simulink model "Frontier40GAPOUT"  (R2015b)
settings: Solver=FixedStepAuto  StartTime=0.0  StopTime=inf  FixedStep=0.1  RelTol=1e-3
values from neighbouring files (symbols this model uses):
  GAPS = []    [ASS.mat]    (also in ENDOFFNC.mat = [26 13 7.5 29.5 29 8.5 29.5 26 30 5.5 34 5 ... (988 elements; FrontierA50GAPSPLOT.m = GAPS_found(i,:); GAPPIE.mat = [26 13 7.5 29.5 29 8.5 29.5 26 30 5.5 34 5 ... (988 elements; HERE.mat = [26 13 7.5 29.5 29 8.5 29.5 26 30 5.5 34 5 ... (988 elements)
  map = [2 0 0 0 0 0 0 0 0 0 0 0 ... (1600 elements, 40x40)]    [INfShitt.mat]
  Method = 1    [ASS.mat]    (also in ENDOFFNC.mat = 0; FrontierA50GAPSPLOT.m = u(end,7); GAPPIE.mat = 0; HERE.mat = 0)
undefined symbols (not defined in the file or in its folder): Data, Data_SL_Info, X, Y, Z
libraries: robotlib x17
settings Model: Creator=einar  LastModifiedBy=einar

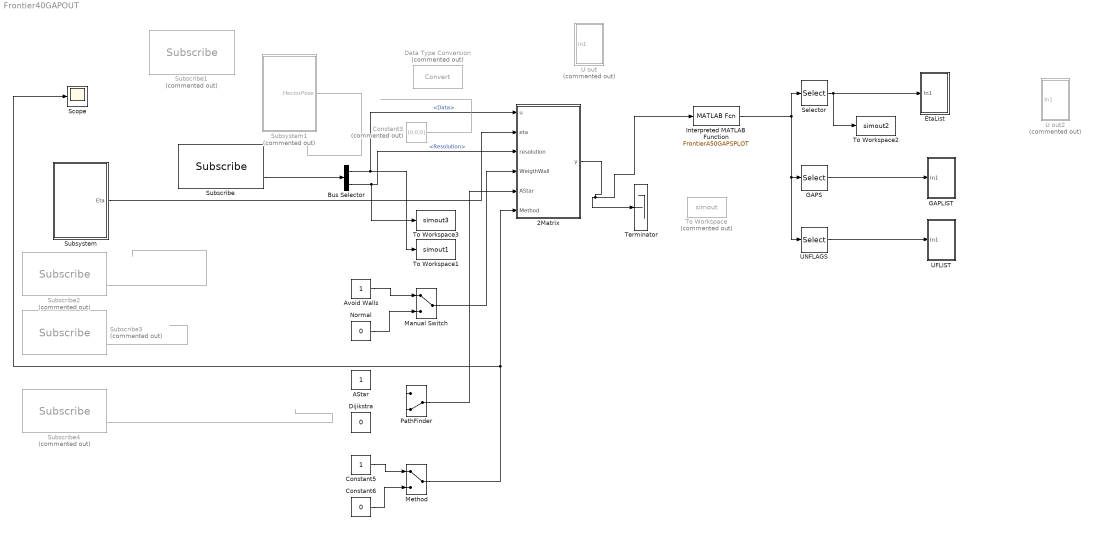
== system Frontier40GAPOUT ==
  2Matrix : MATLAB Function  TreatAsAtomicUnit=on
  AStar : Constant
  Avoid Walls : Constant
  Bus Selector : BusSelector  OutputSignals=Data,Info.Resolution
  Constant3 : Constant  Commented=on  Value=[0;0;0]
  Constant5 : Constant
  Constant6 : Constant  Value=0
  Data Type Conversion : DataTypeConversion  Commented=on
  Dijikstra : Constant  Value=0
  EtaList : Subsystem
  GAPLIST : Subsystem
  GAPS : Selector  InputPortWidth=768  IndexOptions=Index vector (dialog)  Indices=[257:512]  OutputSizes=1
  Interpreted MATLAB Function : MATLABFcn  MATLABFcn=FrontierA50GAPSPLOT  OutputDimensions=768
  Manual Switch : ManualSwitch
  Method : ManualSwitch
  Normal : Constant  Value=0
  PathFinder : ManualSwitch  CurrentSetting=0
  Scope : Scope
  Selector : Selector  InputPortWidth=768  IndexOptions=Index vector (dialog)  Indices=[1:256]  OutputSizes=1
  Subscribe : robotlib/Subscribe  SourceLibraryInfo=This block requires Robotics System Toolbox  topicSource=Select from ROS network  topic=/map  messageType=nav_msgs/OccupancyGrid  sampleTime=0.5  messageQueueLength=1
  Subscribe1 : robotlib/Subscribe  Commented=on  SourceLibraryInfo=This block requires Robotics System Toolbox  topicSource=Select from ROS network  topic=/ExploredOccupancyGrid  messageType=nav_msgs/OccupancyGrid  sampleTime=0.5  messageQueueLength=1
  Subscribe2 : robotlib/Subscribe  Commented=on  SourceLibraryInfo=This block requires Robotics System Toolbox  topicSource=Specify your own  topic=/AStar  messageType=std_msgs/Bool  sampleTime=-1  messageQueueLength=1
  Subscribe3 : robotlib/Subscribe  Commented=on  SourceLibraryInfo=This block requires Robotics System Toolbox  topicSource=Specify your own  topic=/WeighWall  messageType=std_msgs/Bool  sampleTime=-1  messageQueueLength=1
  Subscribe4 : robotlib/Subscribe  Commented=on  SourceLibraryInfo=This block requires Robotics System Toolbox  topicSource=Specify your own  topic=/Method  messageType=std_msgs/Bool  sampleTime=-1  messageQueueLength=1
  Subsystem : Subsystem
  Subsystem1 : Subsystem  Commented=on
  Terminator : Terminator
  To Workspace : ToWorkspace  Commented=on  VariableName=simout  SaveFormat=Timeseries  SampleTime=-1
  To Workspace1 : ToWorkspace  VariableName=simout1  SaveFormat=Timeseries  SampleTime=-1
  To Workspace2 : ToWorkspace  VariableName=simout2  SaveFormat=Timeseries  SampleTime=-1
  To Workspace3 : ToWorkspace  VariableName=simout3  SaveFormat=Timeseries  SampleTime=-1
  U out : Subsystem  Commented=on
  U out2 : Subsystem  Commented=on
  "UFLIST " : Subsystem
  UNFLAGS : Selector  InputPortWidth=768  IndexOptions=Index vector (dialog)  Indices=[513:768]  OutputSizes=1
  wires:
  Subscribe/2 -> Bus Selector/1
  Bus Selector/1 -> To Workspace1/1, 2Matrix/1(u)  "<Data>"
  2Matrix/1(y) -> Interpreted MATLAB Function/1, Terminator/1
  Subsystem/1(Eta) -> 2Matrix/2(eta)
  Subsystem1/1("HectorPose ") -> ?
  Bus Selector/2 -> To Workspace3/1, 2Matrix/3(resolution)  "<Resolution>"
  Interpreted MATLAB Function/1 -> UNFLAGS/1, GAPS/1, Selector/1
  ? -> U out/1(In1)
  Subscribe2/2 -> ?
  Subscribe3/2 -> ?
  Subscribe4/2 -> ?
  Manual Switch/1 -> 2Matrix/4(WeigthWall)
  Constant3/1 -> ?
  Avoid Walls/1 -> Manual Switch/1
  Normal/1 -> Manual Switch/2
  Constant5/1 -> Method/1
  Constant6/1 -> Method/2
  PathFinder/1 -> 2Matrix/5(AStar)
  Method/1 -> 2Matrix/6(Method), Scope/1
  Selector/1 -> EtaList/1(In1), To Workspace2/1
  GAPS/1 -> GAPLIST/1(In1)
  UNFLAGS/1 -> "UFLIST "/1(In1)

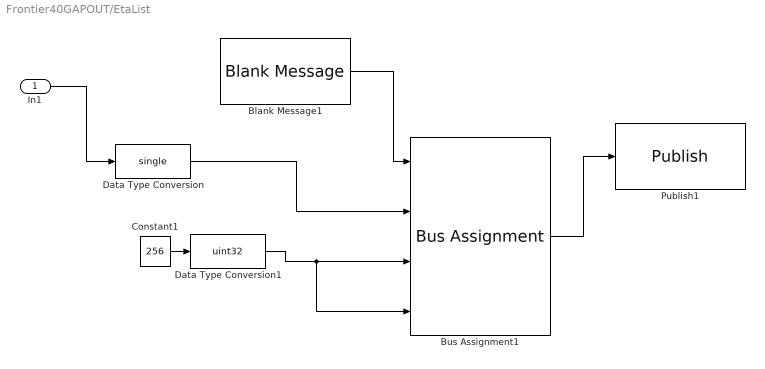
== system Frontier40GAPOUT/EtaList ==
  In1 : Inport
  Blank Message1 : robotlib/Blank Message  SourceLibraryInfo=This block requires Robotics System Toolbox  messageType=std_msgs/Float32MultiArray  SampleTime=inf
  Bus Assignment1 : BusAssignment  AssignedSignals=Data,Data_SL_Info.CurrentLength,Data_SL_Info.ReceivedLength
  Constant1 : Constant  Value=256
  Data Type Conversion : DataTypeConversion  OutDataTypeStr=single
  Data Type Conversion1 : DataTypeConversion  OutDataTypeStr=uint32
  Publish1 : robotlib/Publish  SourceLibraryInfo=This block requires Robotics System Toolbox  topicSource=Specify your own  topic=/EtaSetList  messageType=std_msgs/Float32MultiArray  messageQueueLength=1
  wires:
  Constant1/1 -> Data Type Conversion1/1
  Data Type Conversion/1 -> Bus Assignment1/2
  Bus Assignment1/1 -> Publish1/1
  Blank Message1/1 -> Bus Assignment1/1
  Data Type Conversion1/1 -> Bus Assignment1/4, Bus Assignment1/3
  In1/1 -> Data Type Conversion/1

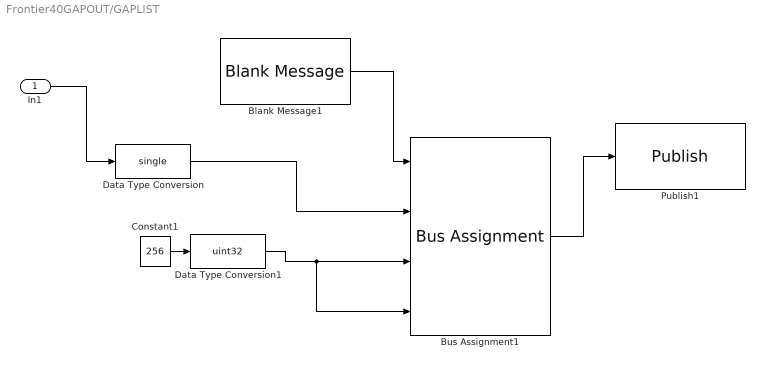
== system Frontier40GAPOUT/GAPLIST ==
  In1 : Inport
  Blank Message1 : robotlib/Blank Message  SourceLibraryInfo=This block requires Robotics System Toolbox  messageType=std_msgs/Float32MultiArray  SampleTime=inf
  Bus Assignment1 : BusAssignment  AssignedSignals=Data,Data_SL_Info.CurrentLength,Data_SL_Info.ReceivedLength
  Constant1 : Constant  Value=256
  Data Type Conversion : DataTypeConversion  OutDataTypeStr=single
  Data Type Conversion1 : DataTypeConversion  OutDataTypeStr=uint32
  Publish1 : robotlib/Publish  SourceLibraryInfo=This block requires Robotics System Toolbox  topicSource=Specify your own  topic=/GAPS  messageType=std_msgs/Float32MultiArray  messageQueueLength=1
  wires:
  In1/1 -> Data Type Conversion/1
  Data Type Conversion1/1 -> Bus Assignment1/3, Bus Assignment1/4
  Blank Message1/1 -> Bus Assignment1/1
  Bus Assignment1/1 -> Publish1/1
  Data Type Conversion/1 -> Bus Assignment1/2
  Constant1/1 -> Data Type Conversion1/1

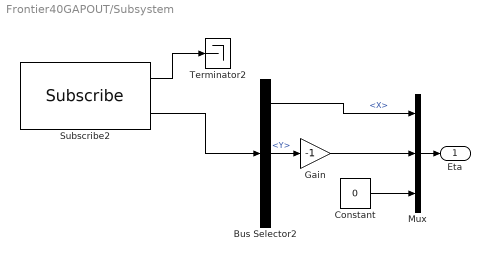
== system Frontier40GAPOUT/Subsystem ==
  Bus Selector2 : BusSelector  OutputSignals=X,Y,Z
  Constant : Constant  Value=0
  Gain : Gain  Gain=-1
  Mux : Mux  Inputs=3
  Subscribe2 : robotlib/Subscribe  SourceLibraryInfo=This block requires Robotics System Toolbox  topicSource=Specify your own  topic=/Eta  messageType=geometry_msgs/Vector3  sampleTime=-1  messageQueueLength=1
  Terminator2 : Terminator
  Eta : Outport
  wires:
  Bus Selector2/1 -> Mux/1  "<X>"
  Subscribe2/2 -> Bus Selector2/1
  Mux/1 -> Eta/1
  Subscribe2/1 -> Terminator2/1
  Bus Selector2/2 -> Gain/1  "<Y>"
  Constant/1 -> Mux/3
  Gain/1 -> Mux/2

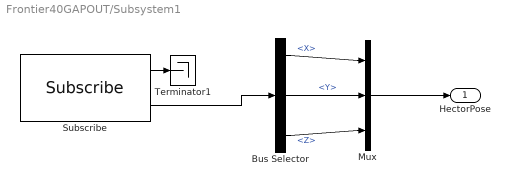
== system Frontier40GAPOUT/Subsystem1 ==
  Bus Selector : BusSelector  OutputSignals=Pose.Pose.Position.X,Pose.Pose.Position.Y,Pose.Pose.Orientation.Z
  Mux : Mux  Inputs=3
  Subscribe : robotlib/Subscribe  SourceLibraryInfo=This block requires Robotics System Toolbox  topicSource=Select from ROS network  topic=/poseupdate  messageType=geometry_msgs/PoseWithCovarianceStamped  sampleTime=-1  messageQueueLength=1
  Terminator1 : Terminator
  "HectorPose " : Outport
  wires:
  Subscribe/2 -> Bus Selector/1
  Subscribe/1 -> Terminator1/1
  Bus Selector/3 -> Mux/3  "<Z>"
  Bus Selector/2 -> Mux/2  "<Y>"
  Bus Selector/1 -> Mux/1  "<X>"
  Mux/1 -> "HectorPose "/1

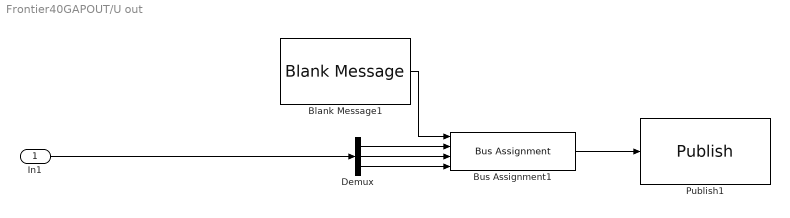
== system Frontier40GAPOUT/U out ==
  In1 : Inport
  Blank Message1 : robotlib/Blank Message  SourceLibraryInfo=This block requires Robotics System Toolbox  messageType=geometry_msgs/Vector3  SampleTime=inf
  Bus Assignment1 : BusAssignment  AssignedSignals=X,Y,Z
  Demux : Demux  Outputs=3
  Publish1 : robotlib/Publish  SourceLibraryInfo=This block requires Robotics System Toolbox  topicSource=Specify your own  topic=/U  messageType=geometry_msgs/Vector3  messageQueueLength=1
  wires:
  Bus Assignment1/1 -> Publish1/1
  Blank Message1/1 -> Bus Assignment1/1
  In1/1 -> Demux/1
  Demux/1 -> Bus Assignment1/2
  Demux/2 -> Bus Assignment1/3
  Demux/3 -> Bus Assignment1/4

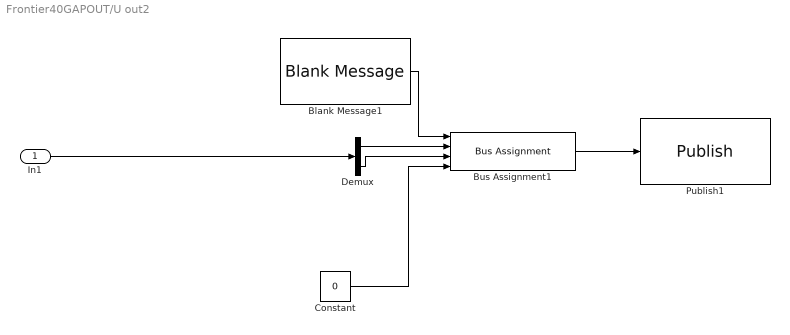
== system Frontier40GAPOUT/U out2 ==
  In1 : Inport
  Blank Message1 : robotlib/Blank Message  SourceLibraryInfo=This block requires Robotics System Toolbox  messageType=geometry_msgs/Vector3  SampleTime=inf
  Bus Assignment1 : BusAssignment  AssignedSignals=X,Y,Z
  Constant : Constant  Value=0
  Demux : Demux  Outputs=2
  Publish1 : robotlib/Publish  SourceLibraryInfo=This block requires Robotics System Toolbox  topicSource=Select from ROS network  topic=/EtaSet  messageType=geometry_msgs/Vector3  messageQueueLength=1
  wires:
  Bus Assignment1/1 -> Publish1/1
  Blank Message1/1 -> Bus Assignment1/1
  In1/1 -> Demux/1
  Demux/1 -> Bus Assignment1/2
  Demux/2 -> Bus Assignment1/3
  Constant/1 -> Bus Assignment1/4

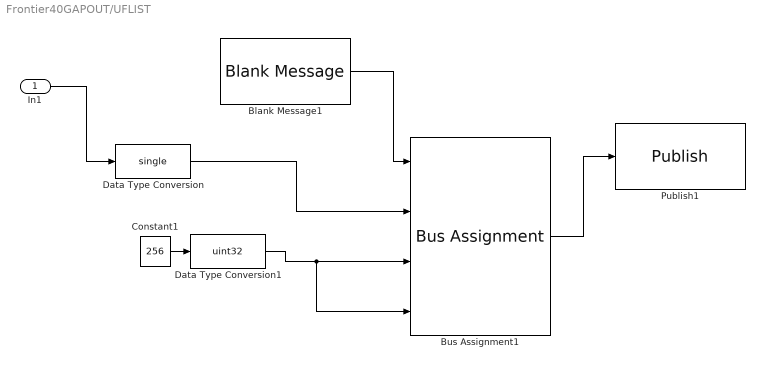
== system Frontier40GAPOUT/UFLIST  ==
  In1 : Inport
  Blank Message1 : robotlib/Blank Message  SourceLibraryInfo=This block requires Robotics System Toolbox  messageType=std_msgs/Float32MultiArray  SampleTime=inf
  Bus Assignment1 : BusAssignment  AssignedSignals=Data,Data_SL_Info.CurrentLength,Data_SL_Info.ReceivedLength
  Constant1 : Constant  Value=256
  Data Type Conversion : DataTypeConversion  OutDataTypeStr=single
  Data Type Conversion1 : DataTypeConversion  OutDataTypeStr=uint32
  Publish1 : robotlib/Publish  SourceLibraryInfo=This block requires Robotics System Toolbox  topicSource=Specify your own  topic=/UNFGAPS  messageType=std_msgs/Float32MultiArray  messageQueueLength=1
  wires:
  Constant1/1 -> Data Type Conversion1/1
  Data Type Conversion/1 -> Bus Assignment1/2
  Bus Assignment1/1 -> Publish1/1
  Blank Message1/1 -> Bus Assignment1/1
  Data Type Conversion1/1 -> Bus Assignment1/4, Bus Assignment1/3
  In1/1 -> Data Type Conversion/1

== matlab function Frontier40GAPOUT/2Matrix ==
  data: u input; y output; eta input; resolution input; WeigthWall input; AStar input; Method input
function y  = fcn(u,eta,resolution,WeigthWall,AStar,Method)
K=length(u)^0.5;
y=zeros(K+1,K);
MAP=zeros(K+1,K)
for i=1:K;
    MAP(i,1:K)=u((i-1)*K+1:i*K);
end
MAP(K+1,1:3)=eta;
MAP(K+1,4)=resolution;
MAP(K+1,5)=WeigthWall;
MAP(K+1,6)=AStar;
MAP(K+1,7)=Method;
Method=Method

y = (MAP);
